simulink model "non_lin_6_DOF"  (R2021b)
settings: Solver=VariableStepAuto  StartTime=0.0  StopTime=Inf  RelTol=1e-3
values from neighbouring files (symbols this model uses):
  u1max = 25*pi/180    (= 0.436332312999)    [RunSecond_initCode.m]    (also in workspacedat.mat = 0.261799387799)
  u1min = -25*pi/180    (= -0.436332312999)    [RunSecond_initCode.m]    (also in workspacedat.mat = -0.523598775598)
  u2max = 25*pi/180    (= 0.436332312999)    [RunSecond_initCode.m]    (also in workspacedat.mat = 0.349065850399)
  u2min = -25*pi/180    (= -0.436332312999)    [RunSecond_initCode.m]    (also in workspacedat.mat = -0.488692190558)
  u3max = 25*pi/180    (= 0.436332312999)    [RunSecond_initCode.m]    (also in workspacedat.mat = 0.453785605519)
  u3min = -25*pi/180    (= -0.436332312999)    [RunSecond_initCode.m]    (also in workspacedat.mat = -0.453785605519)
  u4max = 75*pi/180    (= 1.308996939)    [RunSecond_initCode.m]    (also in workspacedat.mat)
  u4min = -5*pi/180    (= -0.0872664625997)    [RunSecond_initCode.m]    (also in workspacedat.mat)
  u5max = 75*pi/180    (= 1.308996939)    [RunSecond_initCode.m]    (also in workspacedat.mat)
  u5min = -5*pi/180    (= -0.0872664625997)    [RunSecond_initCode.m]    (also in workspacedat.mat)
  x0 = [85; 0; 0; 0; 0; 0; 0; 0.1; 0]    [RunSecond_initCode.m]    (also in workspacedat.mat = [85 0 0 0 0 0 0 0.1 0])
undefined symbols (not defined in the file or in its folder): nav_eqn, NonLin6DOFModel
libraries: aerolibfltsims x2, simulink_extras x2, aerolibutil x2, aerolibanimutils x1, vrlib x1
settings Model: Creator=Abi  LastModifiedBy=Abi

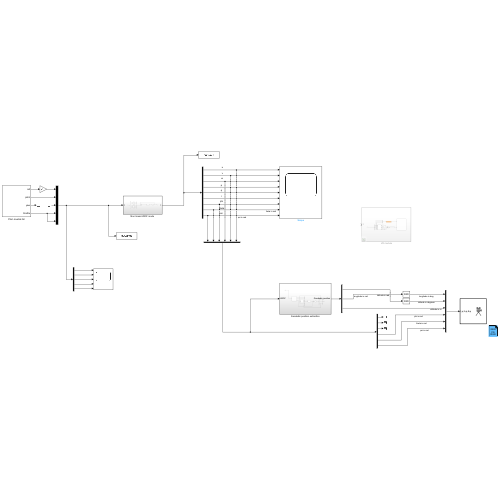
[thumbnail: Simulink's stored preview of the top-level diagram]
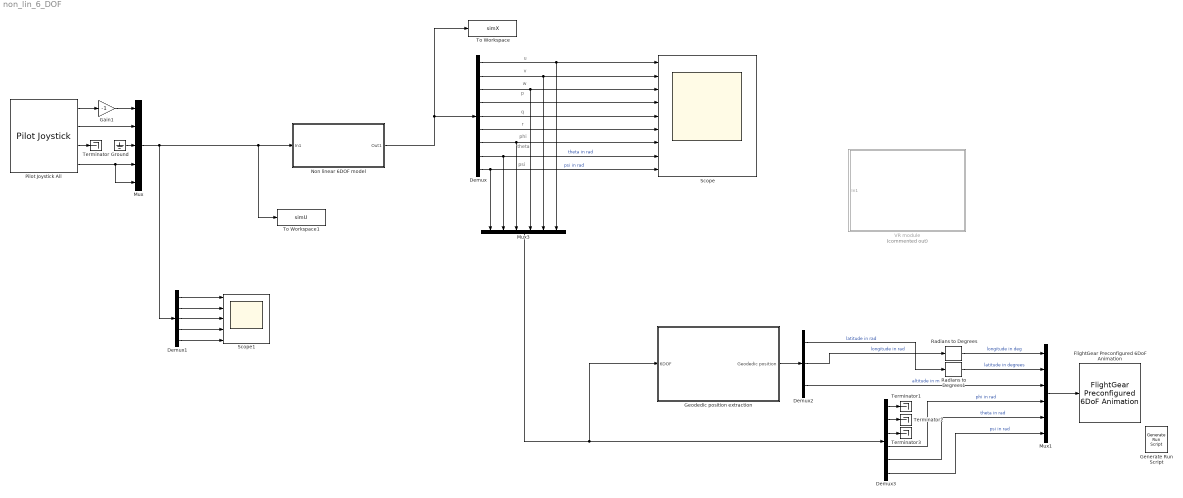
== system non_lin_6_DOF ==
  note: psi
  note: theta
  note: phi
  note: r
  note: q
  note: p
  note: w
  note: v
  note: u
  Demux : Demux  Outputs=9
  Demux1 : Demux  Outputs=5
  Demux2 : Demux  Outputs=3
  Demux3 : Demux  Outputs=6
  FlightGear Preconfigured 6DoF Animation : aerolibfltsims/FlightGear Preconfigured 6DoF Animation  xFlightGearVersion=v2019.1  DestinationIpAddress=127.0.0.1  DestinationPort=5502  SampleTime=1/30  packetVersion=24
  Gain1 : Gain  Gain=-1
  Generate Run Script : aerolibfltsims/Generate Run Script  Architecture=Win64  dataFlow=Send  GeometryModelName=c172p  AirportId=KSFO  RunwayId=10L  InitialAltitude=7224  InitialHeading=113  OffsetDistance=4.72  OffsetAzimuth=0  InstallScenery=off  DisableShaders=on  OriginAddress=127.0.0.1  DestinationPort=5502  OriginPort=5505  LocalAddress=127.0.0.1  OutputFileName=runfg.bat  FlightGearBaseDirectory=C:\Program Files\FlightGear 2020.3
  Geodedic position extraction : Subsystem
  Ground : Ground
  Mux : Mux  Inputs=5
  Mux1 : Mux  Inputs=6
  Mux3 : Mux  Inputs=6
  Non linear 6DOF model : Subsystem
  Pilot Joystick All : aerolibanimutils/Pilot Joystick  JoystickID=Joystick1  OutputConfiguration=FourAxis  SampleTime=1/30
  Radians to Degrees : simulink_extras/Transformations/Radians to Degrees
  Radians to Degrees1 : simulink_extras/Transformations/Radians to Degrees
  Scope : Scope  NumInputPorts=9
  Scope1 : Scope  NumInputPorts=5
  Terminator{,1..3} (4 alike) : Terminator
  To Workspace : ToWorkspace  VariableName=simX  SaveFormat=Timeseries  SampleTime=-1
  To Workspace1 : ToWorkspace  VariableName=simU  SaveFormat=Timeseries  SampleTime=-1
  VR module : Subsystem  Commented=on
  wires:
  Non linear 6DOF model/1(Out1) -> Demux/1, To Workspace/1
  Mux/1 -> Demux1/1, Non linear 6DOF model/1(In1), To Workspace1/1
  Demux/4 -> Scope/4
  Demux/5 -> Scope/5
  Demux/6 -> Scope/6
  Pilot Joystick All/2 -> Mux/2
  Pilot Joystick All/4 -> Mux/5, Mux/4
  Demux/3 -> Scope/3, Mux3/4
  Demux/2 -> Mux3/5, Scope/2
  Demux/1 -> Mux3/6, Scope/1
  Pilot Joystick All/3 -> Terminator/1
  Ground/1 -> Mux/3
  Demux1/3 -> Scope1/3
  Demux1/2 -> Scope1/2
  Demux1/1 -> Scope1/1
  Demux1/4 -> Scope1/4
  Demux1/5 -> Scope1/5
  Pilot Joystick All/1 -> Gain1/1
  Gain1/1 -> Mux/1
  Demux/7 -> Scope/7, Mux3/3
  Demux/8 -> Mux3/2, Scope/8  "theta in rad"
  Demux/9 -> Mux3/1, Scope/9  "psi in rad"
  Mux3/1 -> Geodedic position extraction/1(6DOF), Demux3/1
  Geodedic position extraction/1(Geodedic position) -> Demux2/1
  Demux3/2 -> Terminator2/1
  Mux1/1 -> FlightGear Preconfigured 6DoF Animation/1
  Demux3/3 -> Terminator3/1
  Demux3/6 -> Mux1/6  "psi in rad"
  Demux2/3 -> Mux1/3  "altitude in m"
  Demux2/2 -> Radians to Degrees/1  "longitude in rad"
  Radians to Degrees1/1 -> Mux1/2  "latitude in degrees"
  Demux3/5 -> Mux1/5  "theta in rad"
  Demux3/4 -> Mux1/4  "phi in rad"
  Demux2/1 -> Radians to Degrees1/1  "latitude in rad"
  Demux3/1 -> Terminator1/1
  Radians to Degrees/1 -> Mux1/1  "longitude in deg"

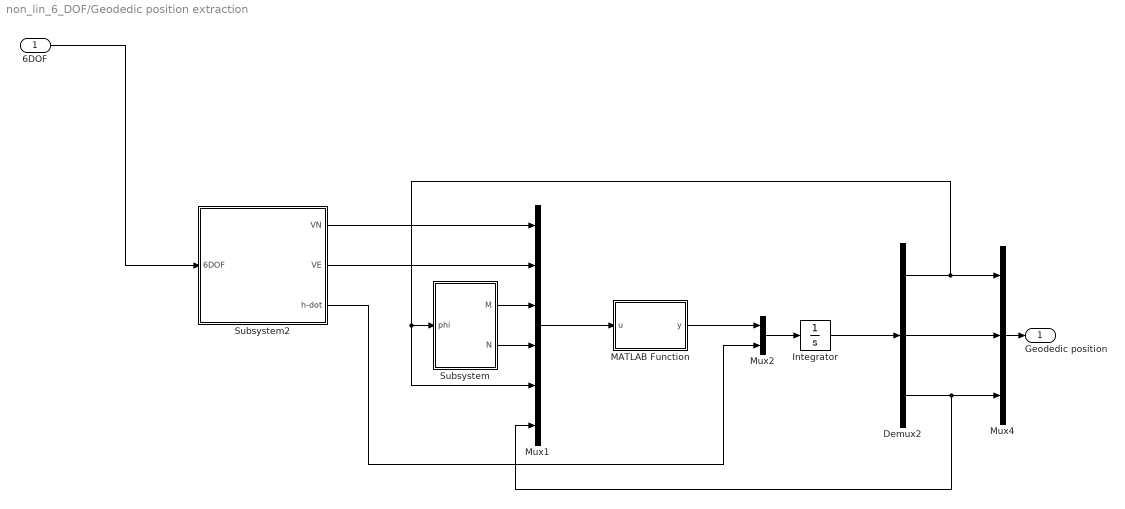
== system non_lin_6_DOF/Geodedic position extraction ==
  6DOF : Inport
  Demux2 : Demux  Outputs=3
  Integrator : Integrator
  MATLAB Function : MATLAB Function  TreatAsAtomicUnit=on
  Mux1 : Mux  Inputs=6
  Mux2 : Mux  Inputs=2
  Mux4 : Mux  Inputs=3
  Subsystem : Subsystem
  Subsystem2 : Subsystem
  Geodedic position : Outport
  wires:
  MATLAB Function/1(y) -> Mux2/1
  Demux2/1 -> Subsystem/1(phi), Mux1/5, Mux4/1
  Mux1/1 -> MATLAB Function/1(u)
  Subsystem2/2(VE) -> Mux1/2
  Subsystem/1(M) -> Mux1/3
  Demux2/3 -> Mux1/6, Mux4/3
  Mux4/1 -> Geodedic position/1
  Integrator/1 -> Demux2/1
  Subsystem2/1(VN) -> Mux1/1
  Subsystem/2(N) -> Mux1/4
  Mux2/1 -> Integrator/1
  Subsystem2/3(h-dot) -> Mux2/2
  Demux2/2 -> Mux4/2
  6DOF/1 -> Subsystem2/1(6DOF)

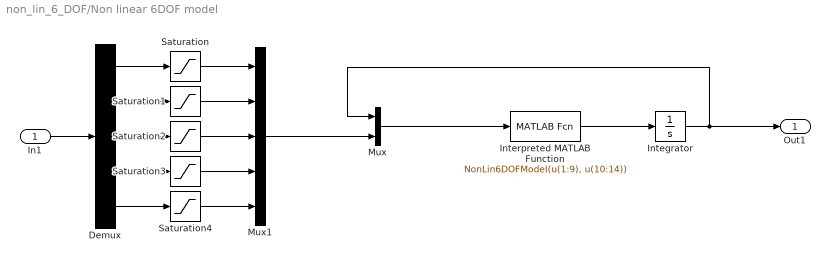
== system non_lin_6_DOF/Non linear 6DOF model ==
  In1 : Inport
  Demux : Demux  Outputs=5
  Integrator : Integrator  InitialCondition=x0
  Interpreted MATLAB Function : MATLABFcn  MATLABFcn=NonLin6DOFModel(u(1:9), u(10:14))  OutputDimensions=9
  Mux : Mux  Inputs=2
  Mux1 : Mux  Inputs=5
  Saturation : Saturate  UpperLimit=u1max  LowerLimit=u1min
  Saturation1 : Saturate  UpperLimit=u2max  LowerLimit=u2min
  Saturation2 : Saturate  UpperLimit=u3max  LowerLimit=u3min
  Saturation3 : Saturate  UpperLimit=u4max  LowerLimit=u4min
  Saturation4 : Saturate  UpperLimit=u5max  LowerLimit=u5min
  Out1 : Outport
  wires:
  Integrator/1 -> Mux/1, Out1/1
  Mux/1 -> Interpreted MATLAB Function/1
  Interpreted MATLAB Function/1 -> Integrator/1
  In1/1 -> Demux/1
  Demux/1 -> Saturation/1
  Demux/2 -> Saturation1/1
  Demux/3 -> Saturation2/1
  Demux/5 -> Saturation4/1
  Demux/4 -> Saturation3/1
  Saturation/1 -> Mux1/1
  Saturation1/1 -> Mux1/2
  Saturation2/1 -> Mux1/3
  Saturation3/1 -> Mux1/4
  Saturation4/1 -> Mux1/5
  Mux1/1 -> Mux/2

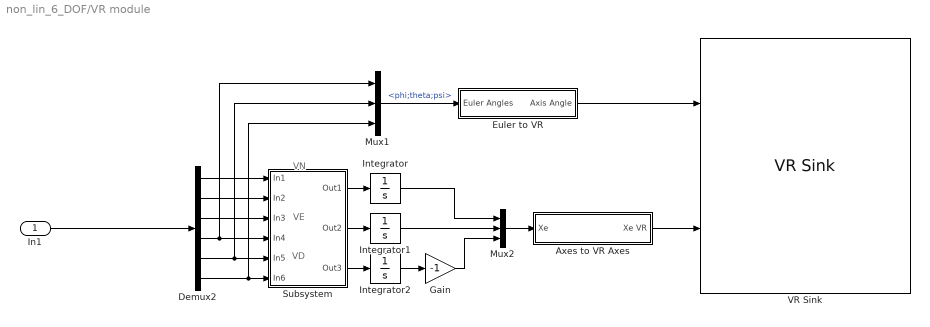
== system non_lin_6_DOF/VR module ==
  note: VD
  note: VE
  note: VN
  In1 : Inport
  Axes to VR Axes : Subsystem
  Demux2 : Demux  Outputs=6
  Euler to VR : Subsystem
  Gain : Gain  Gain=-1
  Integrator : Integrator
  Integrator1 : Integrator
  Integrator2 : Integrator
  Mux1 : Mux  Inputs=3
  Mux2 : Mux  Inputs=3
  Subsystem : Subsystem
  VR Sink : vrlib/VR Sink  InstantiateOnLoad=on  SampleTime=0.1  ViewEnable=on  RemoteChange=off  RemoteView=off  FieldsWritten=HL20.rotation.4.1.1.double#HL20.translation.3.1.1.double  WorldFileName=aeroblk_HL20.wrl  WorldDescription=aeroblk_HL20  AutoView=on  VideoDimensions=[]  AllowVariableSize=off
  wires:
  Subsystem/2(Out2) -> Integrator1/1
  Gain/1 -> Mux2/3
  Axes to VR Axes/1(Xe VR) -> VR Sink/2
  Integrator2/1 -> Gain/1
  Integrator1/1 -> Mux2/2
  Demux2/4 -> Mux1/1, Subsystem/4(In4)
  Mux1/1 -> Euler to VR/1(Euler Angles)  "<phi;theta;psi>"
  Demux2/3 -> Subsystem/3(In3)
  Integrator/1 -> Mux2/1
  Demux2/6 -> Mux1/3, Subsystem/6(In6)
  Euler to VR/1(Axis Angle) -> VR Sink/1
  Demux2/5 -> Mux1/2, Subsystem/5(In5)
  Mux2/1 -> Axes to VR Axes/1(Xe)
  Subsystem/3(Out3) -> Integrator2/1
  Subsystem/1(Out1) -> Integrator/1
  Demux2/2 -> Subsystem/2(In2)
  Demux2/1 -> Subsystem/1(In1)
  In1/1 -> Demux2/1

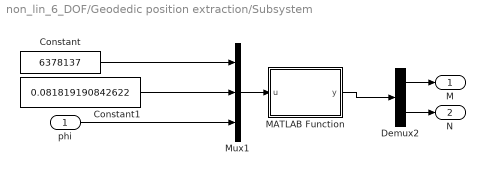
== system non_lin_6_DOF/Geodedic position extraction/Subsystem ==
  phi : Inport
  Constant : Constant  Value=6378137
  Constant1 : Constant  Value=0.081819190842622
  Demux2 : Demux  Outputs=2
  MATLAB Function : MATLAB Function  TreatAsAtomicUnit=on
  Mux1 : Mux  Inputs=3
  M : Outport
  N : Outport  Port=2
  wires:
  Mux1/1 -> MATLAB Function/1(u)
  Constant1/1 -> Mux1/2
  Constant/1 -> Mux1/1
  Demux2/1 -> M/1
  MATLAB Function/1(y) -> Demux2/1
  phi/1 -> Mux1/3
  Demux2/2 -> N/1

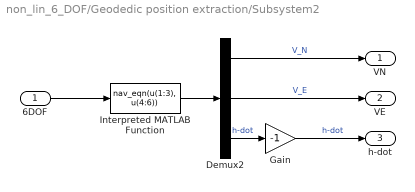
== system non_lin_6_DOF/Geodedic position extraction/Subsystem2 ==
  6DOF : Inport
  Demux2 : Demux  Outputs=3
  Gain : Gain  Gain=-1
  Interpreted MATLAB Function : MATLABFcn  MATLABFcn=nav_eqn(u(1:3), u(4:6))
  VN : Outport
  VE : Outport  Port=2
  h-dot : Outport  Port=3
  wires:
  Demux2/1 -> VN/1  "V_N"
  Gain/1 -> h-dot/1  "h-dot"
  6DOF/1 -> Interpreted MATLAB Function/1
  Demux2/2 -> VE/1  "V_E"
  Demux2/3 -> Gain/1  "h-dot"
  Interpreted MATLAB Function/1 -> Demux2/1

== system non_lin_6_DOF/VR module/Axes to VR Axes ==
  Xe : Inport
  Concatenate : Concatenate  NumInputs=3
  Demux : Demux  Outputs=3
      settings: DisplayOption=none
  rad-->deg : Gain  Gain=-1  SaturateOnIntegerOverflow=on  OutDataTypeStr=Inherit: Same as input  ParamDataTypeStr=Inherit: Same as input
  rad-->deg1 : Gain  Gain=-1  SaturateOnIntegerOverflow=on  OutDataTypeStr=Inherit: Same as input  ParamDataTypeStr=Inherit: Same as input
  Xe VR : Outport  VectorParamsAs1DForOutWhenUnconnected=off
  wires:
  Xe/1 -> Demux/1
  Demux/1 -> Concatenate/1
  Demux/2 -> rad-->deg/1
  Demux/3 -> rad-->deg1/1
  Concatenate/1 -> Xe VR/1
  rad-->deg1/1 -> Concatenate/2
  rad-->deg/1 -> Concatenate/3

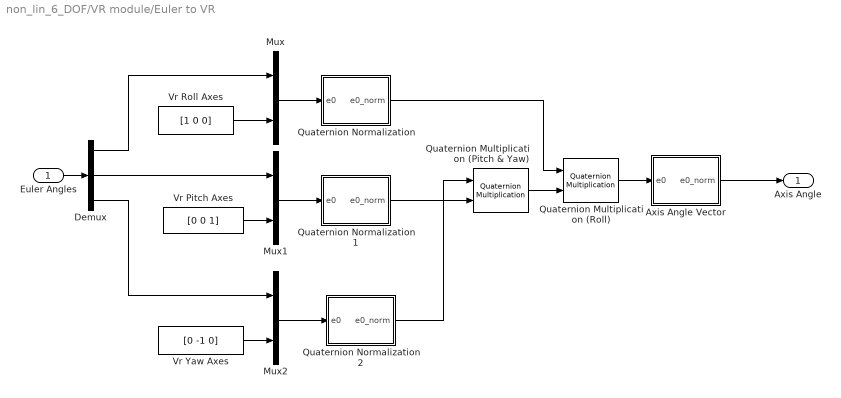
== system non_lin_6_DOF/VR module/Euler to VR ==
  Euler Angles : Inport
  Axis Angle Vector : Subsystem
  Demux : Demux  Outputs=3
      settings: DisplayOption=none
  Mux : Mux  Inputs=2
  Mux1 : Mux  Inputs=2
  Mux2 : Mux  Inputs=2
  Quaternion Multiplication (Pitch & Yaw) : aerolibutil/Quaternion Multiplication
  Quaternion Multiplication (Roll) : aerolibutil/Quaternion Multiplication
  Quaternion Normalization : Subsystem
  Quaternion Normalization1 : Subsystem
  Quaternion Normalization2 : Subsystem
  Vr Pitch Axes : Constant  Value=[0 0 1]
  Vr Roll Axes : Constant  Value=[1 0 0]
  Vr Yaw Axes : Constant  Value=[0 -1 0]
  Axis Angle : Outport  VectorParamsAs1DForOutWhenUnconnected=off
  wires:
  Quaternion Multiplication (Roll)/1 -> Axis Angle Vector/1(e0)
  Quaternion Multiplication (Pitch & Yaw)/1 -> Quaternion Multiplication (Roll)/2
  Axis Angle Vector/1(e0_norm) -> Axis Angle/1
  Quaternion Normalization/1(e0_norm) -> Quaternion Multiplication (Roll)/1
  Quaternion Normalization2/1(e0_norm) -> Quaternion Multiplication (Pitch & Yaw)/1
  Quaternion Normalization1/1(e0_norm) -> Quaternion Multiplication (Pitch & Yaw)/2
  Mux2/1 -> Quaternion Normalization2/1(e0)
  Mux1/1 -> Quaternion Normalization1/1(e0)
  Mux/1 -> Quaternion Normalization/1(e0)
  Demux/3 -> Mux2/1
  Vr Yaw Axes/1 -> Mux2/2
  Demux/2 -> Mux1/1
  Vr Pitch Axes/1 -> Mux1/2
  Demux/1 -> Mux/1
  Vr Roll Axes/1 -> Mux/2
  Euler Angles/1 -> Demux/1

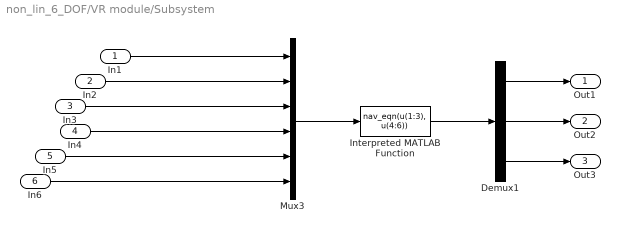
== system non_lin_6_DOF/VR module/Subsystem ==
  In1 : Inport
  In2 : Inport  Port=2
  In3 : Inport  Port=3
  In4 : Inport  Port=4
  In5 : Inport  Port=5
  In6 : Inport  Port=6
  Demux1 : Demux  Outputs=3
  Interpreted MATLAB Function : MATLABFcn  MATLABFcn=nav_eqn(u(1:3), u(4:6))
  Mux3 : Mux  Inputs=6
  Out1 : Outport
  Out2 : Outport  Port=2
  Out3 : Outport  Port=3
  wires:
  In2/1 -> Mux3/2
  In6/1 -> Mux3/6
  Demux1/3 -> Out3/1
  Demux1/2 -> Out2/1
  Mux3/1 -> Interpreted MATLAB Function/1
  Interpreted MATLAB Function/1 -> Demux1/1
  In4/1 -> Mux3/4
  In1/1 -> Mux3/1
  In3/1 -> Mux3/3
  Demux1/1 -> Out1/1
  In5/1 -> Mux3/5

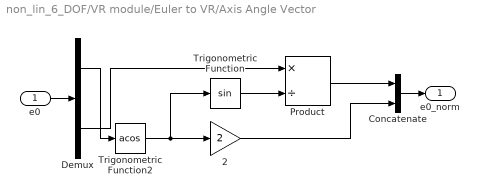
== system non_lin_6_DOF/VR module/Euler to VR/Axis Angle Vector ==
  e0 : Inport
  2 : Gain  Gain=2  SaturateOnIntegerOverflow=on  OutDataTypeStr=Inherit: Same as input  ParamDataTypeStr=Inherit: Same as input
  Concatenate : Concatenate
  Demux : Demux  Outputs=[1 3 ]
      settings: DisplayOption=none
  Product : Product  Inputs=*/  InputSameDT=on  SaturateOnIntegerOverflow=on  OutDataTypeStr=Inherit: Same as first input
  Trigonometric Function : Trigonometry
  Trigonometric Function2 : Trigonometry  Operator=acos
  e0_norm : Outport  VectorParamsAs1DForOutWhenUnconnected=off
  wires:
  Demux/1 -> Trigonometric Function2/1
  Demux/2 -> Product/1
  Concatenate/1 -> e0_norm/1
  Product/1 -> Concatenate/1
  2/1 -> Concatenate/2
  Trigonometric Function/1 -> Product/2
  Trigonometric Function2/1 -> Trigonometric Function/1, 2/1
  e0/1 -> Demux/1

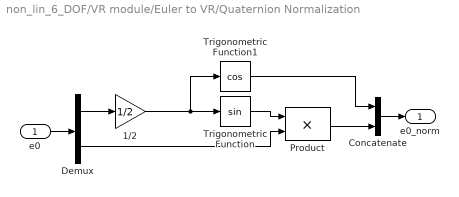
== system non_lin_6_DOF/VR module/Euler to VR/Quaternion Normalization ==
  e0 : Inport
  1/2 : Gain  Gain=1/2  SaturateOnIntegerOverflow=on  OutDataTypeStr=Inherit: Same as input  ParamDataTypeStr=Inherit: Same as input
  Concatenate : Concatenate
  Demux : Demux  Outputs=[1 3]
      settings: DisplayOption=none
  Product : Product  InputSameDT=on  SaturateOnIntegerOverflow=on  OutDataTypeStr=Inherit: Same as first input
  Trigonometric Function : Trigonometry
  Trigonometric Function1 : Trigonometry  Operator=cos
  e0_norm : Outport  VectorParamsAs1DForOutWhenUnconnected=off
  wires:
  Trigonometric Function1/1 -> Concatenate/1
  Demux/2 -> Product/2
  Demux/1 -> 1/2/1
  Concatenate/1 -> e0_norm/1
  Product/1 -> Concatenate/2
  Trigonometric Function/1 -> Product/1
  1/2/1 -> Trigonometric Function1/1, Trigonometric Function/1
  e0/1 -> Demux/1

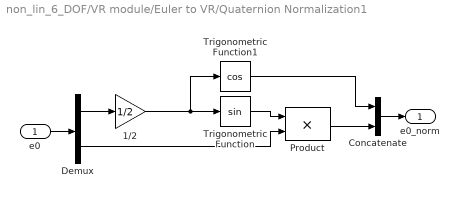
== system non_lin_6_DOF/VR module/Euler to VR/Quaternion Normalization1 ==
  e0 : Inport
  1/2 : Gain  Gain=1/2  SaturateOnIntegerOverflow=on  OutDataTypeStr=Inherit: Same as input  ParamDataTypeStr=Inherit: Same as input
  Concatenate : Concatenate
  Demux : Demux  Outputs=[1 3]
      settings: DisplayOption=none
  Product : Product  InputSameDT=on  SaturateOnIntegerOverflow=on  OutDataTypeStr=Inherit: Same as first input
  Trigonometric Function : Trigonometry
  Trigonometric Function1 : Trigonometry  Operator=cos
  e0_norm : Outport  VectorParamsAs1DForOutWhenUnconnected=off
  wires:
  e0/1 -> Demux/1
  1/2/1 -> Trigonometric Function/1, Trigonometric Function1/1
  Trigonometric Function/1 -> Product/1
  Product/1 -> Concatenate/2
  Concatenate/1 -> e0_norm/1
  Demux/1 -> 1/2/1
  Demux/2 -> Product/2
  Trigonometric Function1/1 -> Concatenate/1

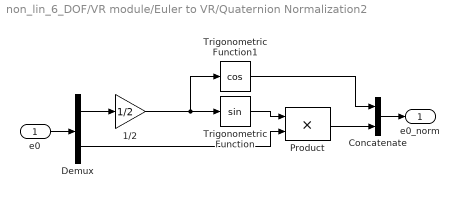
== system non_lin_6_DOF/VR module/Euler to VR/Quaternion Normalization2 ==
  e0 : Inport
  1/2 : Gain  Gain=1/2  SaturateOnIntegerOverflow=on  OutDataTypeStr=Inherit: Same as input  ParamDataTypeStr=Inherit: Same as input
  Concatenate : Concatenate
  Demux : Demux  Outputs=[1 3]
      settings: DisplayOption=none
  Product : Product  InputSameDT=on  SaturateOnIntegerOverflow=on  OutDataTypeStr=Inherit: Same as first input
  Trigonometric Function : Trigonometry
  Trigonometric Function1 : Trigonometry  Operator=cos
  e0_norm : Outport  VectorParamsAs1DForOutWhenUnconnected=off
  wires:
  Trigonometric Function1/1 -> Concatenate/1
  Demux/2 -> Product/2
  Demux/1 -> 1/2/1
  Concatenate/1 -> e0_norm/1
  Product/1 -> Concatenate/2
  Trigonometric Function/1 -> Product/1
  1/2/1 -> Trigonometric Function1/1, Trigonometric Function/1
  e0/1 -> Demux/1

== matlab function non_lin_6_DOF/Geodedic position extraction/Subsystem/MATLAB Function ==
  data: u input; y output
function y = fcn(u)
%#codegen
M = u(1)*(1-(u(2)^2))/(1-(u(2)^2)*(sin(u(3)^2)))^(3/2);
N = u(1)/(1-(u(2)^2)*(sin(u(3)^2)))^(1/2);
y = [M; N];

== matlab function non_lin_6_DOF/Geodedic position extraction/MATLAB Function ==
  data: u input; y output
function y = fcn(u)
phi_dot = u(1)/(u(3)+u(6)); 
lambda_dot = u(2)/((u(4)+u(6))*cos(u(5)));
y = [phi_dot; lambda_dot];
